simulink library "state_to_relay"  (R2024b)
settings: Solver=VariableStepAuto  StartTime=0.0  StopTime=10.0  RelTol=1e-3
settings Model: Creator=mainuser  LastModifiedBy=mainuser

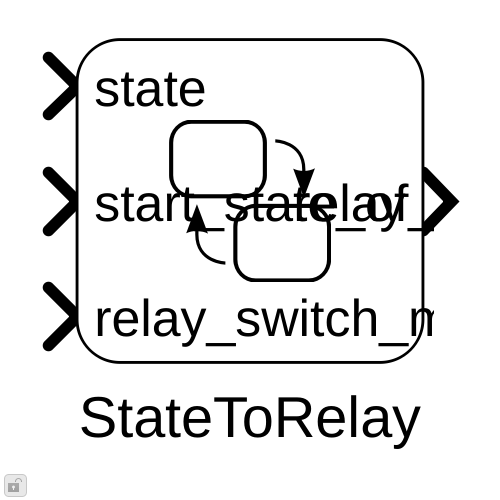
[thumbnail: Simulink's stored preview of the top-level diagram]
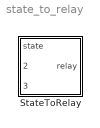
== system state_to_relay ==
  StateToRelay : Stateflow chart  TreatAsAtomicUnit=on

== stateflow chart state_to_relay/StateToRelay ==
  state Change
    relay=true;
  state Init
  state Stay
    relay=false;
  (default) -> Init
  Init -> Change [order 1] : [start_state_of_relay~=state]
  Init -> Stay [order 2]
  Stay -> Change : [hasChanged(state)]
  Change -> Stay : after(relay_switch_ms,msec)
  data: state input boolean size=1; relay output boolean size=1; start_state_of_relay input boolean size=1; relay_switch_ms input uint32 size=1
